simulink library "INT_Rail_PresPeakLim"  (R2016b)
settings: Solver=VariableStepAuto  StartTime=0.0  StopTime=10.0  RelTol=1e-3
settings Model: Creator=Administrator  LastModifiedBy=Administrator

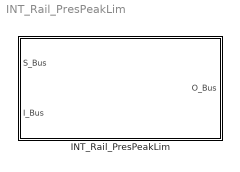
== system INT_Rail_PresPeakLim ==
  INT_Rail_PresPeakLim : Subsystem

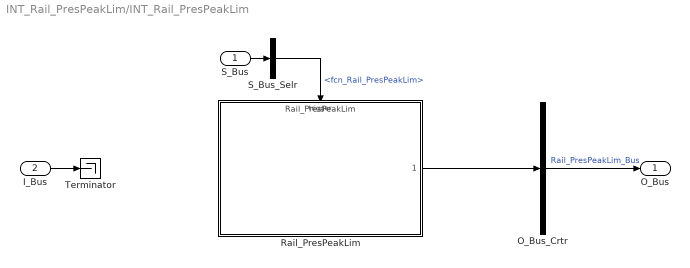
== system INT_Rail_PresPeakLim/INT_Rail_PresPeakLim ==
  S_Bus : Inport
  I_Bus : Inport  Port=2
  O_Bus_Crtr : BusCreator  Inputs=1
  Rail_PresPeakLim : ModelReference  ModelNameDialog=Rail_PresPeakLim  SimulationMode=Normal  ModelReferenceVersion=1.3  TriggerPortName=function  TriggerPortTriggerType=function-call  TriggerPortStatesWhenEnabling=held
  S_Bus_Selr : BusSelector  OutputSignals=fcn_Rail_PresPeakLim
  Terminator : Terminator
  O_Bus : Outport
  wires:
  S_Bus_Selr/1 -> Rail_PresPeakLim/Trigger  "<fcn_Rail_PresPeakLim>"
  S_Bus/1 -> S_Bus_Selr/1
  I_Bus/1 -> Terminator/1
  O_Bus_Crtr/1 -> O_Bus/1  "Rail_PresPeakLim_Bus"
  Rail_PresPeakLim/1 -> O_Bus_Crtr/1
